simulink library "afrt"  (Simulink 8.1)
settings: Solver=ode1  StartTime=0.0  StopTime=Inf  FixedStep=0.001  RelTol=1e-3
PostLoadFcn:
  | , if any(exist('dsrtsu_mdlpostloadfcn', 'file') == [2, 3, 6]), try dsrtsu_mdlpostloadfcn('Execute', bdroot); catch fprintf('Error in PostLoadFcn (dsrtsu_mdlpostloadfcn) for model "%s":\n %s\n', bdroot, lasterr); end, end,
undefined symbols (not defined in the file or in its folder): KJUD_AEBActiveDriverDelay_ms, KJUD_AEBAggrDriverDelay_ms, KJUD_AutoBrakingDelay_ms, ZERO_FLOAT
libraries: hcu_lib x1
settings Model: DSRTSU_INTERNAL_RTI_VER=450  DSRTSU_INTERNAL_RTI_TYPE=rti1401  RTICANMMDATA=struct('GeneralSetupData',struct('modelroot','D:\ELN150201_TAIWAN\trunk\AdasDragon\software\sw_development\arch\app\jud','generalsettings',struct('filesettings',struct('destfolder',struct('Name','RTICANMM_FILES','Check',1),'buildfolder',struct('Name','.','Check',1),'AbsDestfolder',struct('Name','D:\ELN150201_TAIWAN\trunk\AdasDragon\software\sw_development\arch\app\jud\RTICANMM_FILES'),'AbsBuildfolder',struct('Name','D:\ELN150201_TAIWAN\trunk\AdasDragon\software\sw_development\arch\app\jud'))),'options',struct('addpaths',1,'rmpaths',1,'addtrcexclusion',logical(1),'cannavigator',struct('checkmonitoring',0),'show_usrtrc',0,'use_usrtrc',0),'advanced',struct('options',[1 1 1 1 1 1 1 1 1 1 1 1 1 1 1 1 1 1 1 1 1 1 1 1 1 1 1 1 1 1 1 1 1 1 1 1 1 1 1 1 1 1 1 1 1 1 1 1 1 1 1 1 1 1 1 1 1 1 1 1 1 1 1 1 1 1 1 1 1 1 1 1 1 1 1 1 1 1 1 1 1 1 1 1 1 1 1 1 1 1 1 1 1 1 1 1 1 1 1 1]),'MPSetup',{{}},'modelname','afrt','block','afrt'))  DSRTSU_INTERNAL_RTIFPGA=40  Creator=tescamilla  LastModifiedBy=AT015555

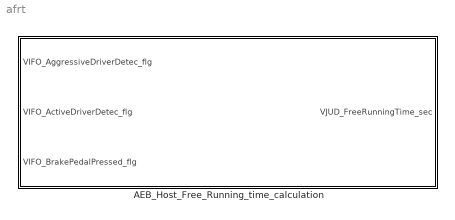
== system afrt ==
  AEB_Host_Free_Running_time_calculation : Subsystem

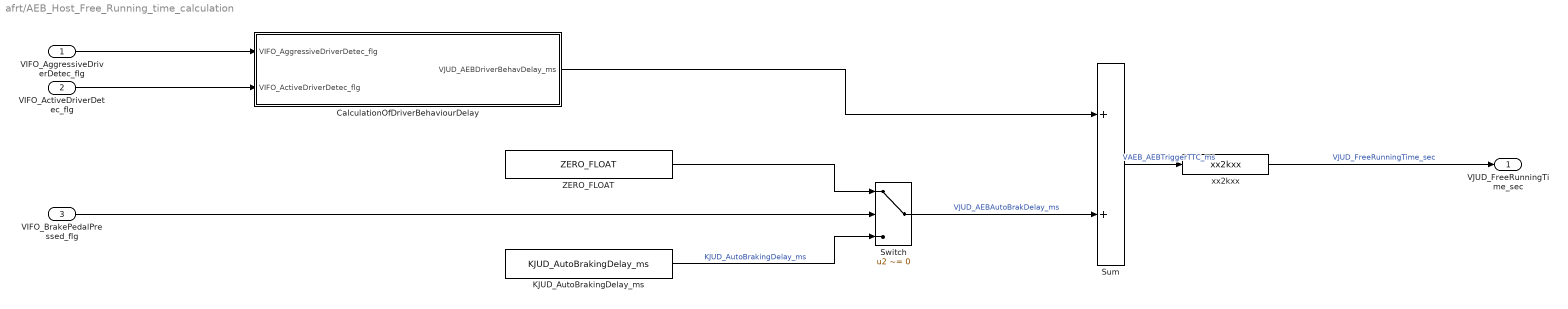
== system afrt/AEB_Host_Free_Running_time_calculation ==
  VIFO_AggressiveDriverDetec_flg : Inport
  VIFO_ActiveDriverDetec_flg : Inport  Port=2
  VIFO_BrakePedalPressed_flg : Inport  Port=3
  CalculationOfDriverBehaviourDelay : Subsystem
  KJUD_AutoBrakingDelay_ms : Constant  Value=KJUD_AutoBrakingDelay_ms  OutDataTypeStr=single
  Sum : Sum
  Switch : Switch  Criteria=u2 ~= 0
  ZERO_FLOAT : Constant  Value=ZERO_FLOAT  OutDataTypeStr=single
  xx2kxx : hcu_lib/xx2kxx
  VJUD_FreeRunningTime_sec : Outport
  wires:
  xx2kxx/1 -> VJUD_FreeRunningTime_sec/1  "VJUD_FreeRunningTime_sec"
  Sum/1 -> xx2kxx/1  "VAEB_AEBTriggerTTC_ms"
  Switch/1 -> Sum/2  "VJUD_AEBAutoBrakDelay_ms"
  VIFO_BrakePedalPressed_flg/1 -> Switch/2
  ZERO_FLOAT/1 -> Switch/1
  VIFO_AggressiveDriverDetec_flg/1 -> CalculationOfDriverBehaviourDelay/1(VIFO_AggressiveDriverDetec_flg)
  KJUD_AutoBrakingDelay_ms/1 -> Switch/3  "KJUD_AutoBrakingDelay_ms"
  VIFO_ActiveDriverDetec_flg/1 -> CalculationOfDriverBehaviourDelay/2(VIFO_ActiveDriverDetec_flg)
  CalculationOfDriverBehaviourDelay/1(VJUD_AEBDriverBehavDelay_ms) -> Sum/1

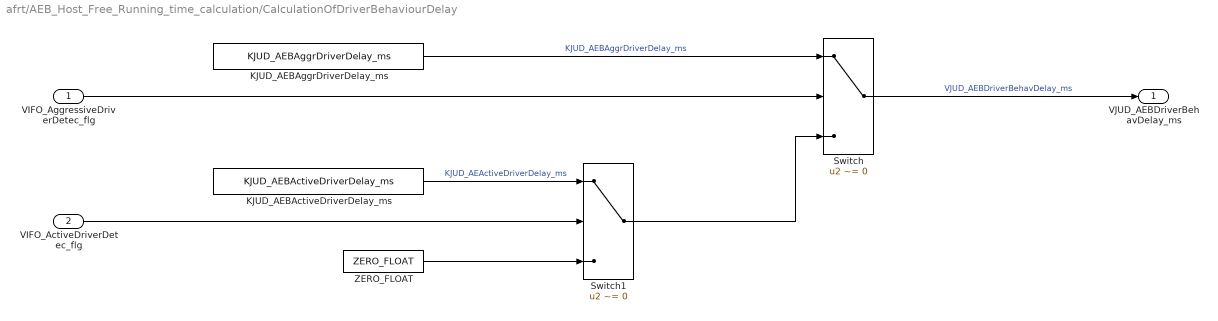
== system afrt/AEB_Host_Free_Running_time_calculation/CalculationOfDriverBehaviourDelay ==
  VIFO_AggressiveDriverDetec_flg : Inport
  VIFO_ActiveDriverDetec_flg : Inport  Port=2
  KJUD_AEBActiveDriverDelay_ms : Constant  Value=KJUD_AEBActiveDriverDelay_ms  OutDataTypeStr=single
  KJUD_AEBAggrDriverDelay_ms : Constant  Value=KJUD_AEBAggrDriverDelay_ms  OutDataTypeStr=single
  Switch : Switch  Criteria=u2 ~= 0
  Switch1 : Switch  Criteria=u2 ~= 0
  ZERO_FLOAT : Constant  Value=ZERO_FLOAT  OutDataTypeStr=single
  VJUD_AEBDriverBehavDelay_ms : Outport
  wires:
  VIFO_AggressiveDriverDetec_flg/1 -> Switch/2
  VIFO_ActiveDriverDetec_flg/1 -> Switch1/2
  Switch1/1 -> Switch/3
  KJUD_AEBAggrDriverDelay_ms/1 -> Switch/1  "KJUD_AEBAggrDriverDelay_ms"
  KJUD_AEBActiveDriverDelay_ms/1 -> Switch1/1  "KJUD_AEActiveDriverDelay_ms"
  Switch/1 -> VJUD_AEBDriverBehavDelay_ms/1  "VJUD_AEBDriverBehavDelay_ms"
  ZERO_FLOAT/1 -> Switch1/3
